simulink model "Tracking_01"  (R2022b)
settings: Solver=ode4  StartTime=0.0  StopTime=50  FixedStep=1e-3  MaxStep=1e-3  RelTol=1e-3
undefined symbols (not defined in the file or in its folder): OF_b, OF_k1, OF_k2, TT_theta1_init, TT_theta2_init, TT_theta3_init, TT_x_init, TT_y_init, v_sat, w_sat
libraries: simulink x18
settings Model: Creator=david  LastModifiedBy=emanuelevitetta

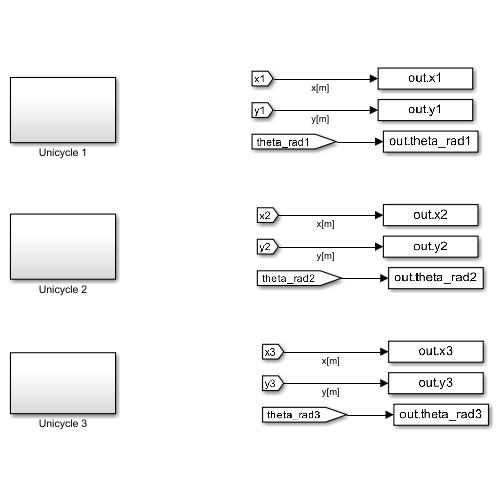
[thumbnail: Simulink's stored preview of the top-level diagram]
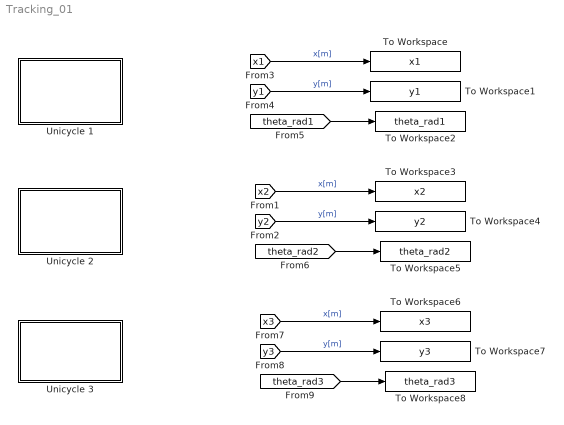
== system Tracking_01 ==
  To Workspace : ToWorkspace  VariableName=x1  SaveFormat=Structure With Time  SampleTime=-1
  To Workspace1 : ToWorkspace  VariableName=y1  SaveFormat=Structure With Time  SampleTime=-1
  To Workspace2 : ToWorkspace  VariableName=theta_rad1  SaveFormat=Structure With Time  SampleTime=-1
  To Workspace3 : ToWorkspace  VariableName=x2  SaveFormat=Structure With Time  SampleTime=-1
  To Workspace4 : ToWorkspace  VariableName=y2  SaveFormat=Structure With Time  SampleTime=-1
  To Workspace5 : ToWorkspace  VariableName=theta_rad2  SaveFormat=Structure With Time  SampleTime=-1
  To Workspace6 : ToWorkspace  VariableName=x3  SaveFormat=Structure With Time  SampleTime=-1
  To Workspace7 : ToWorkspace  VariableName=y3  SaveFormat=Structure With Time  SampleTime=-1
  To Workspace8 : ToWorkspace  VariableName=theta_rad3  SaveFormat=Structure With Time  SampleTime=-1
  Unicycle 1 : Subsystem
  Unicycle 2 : Subsystem
  Unicycle 3 : Subsystem
  wires:
  [x1] -> To Workspace/1  "x[m]"
  [y1] -> To Workspace1/1  "y[m]"
  [theta_rad1] -> To Workspace2/1
  [x2] -> To Workspace3/1  "x[m]"
  [y2] -> To Workspace4/1  "y[m]"
  [theta_rad2] -> To Workspace5/1
  [theta_rad3] -> To Workspace8/1
  [y3] -> To Workspace7/1  "y[m]"
  [x3] -> To Workspace6/1  "x[m]"

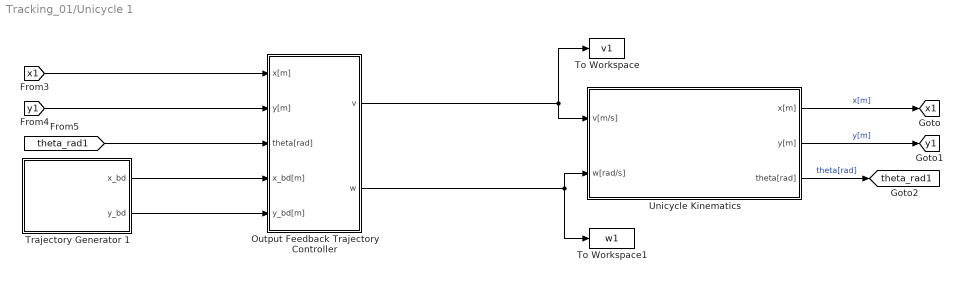
== system Tracking_01/Unicycle 1 ==
  Output Feedback Trajectory Controller : Subsystem
  To Workspace : ToWorkspace  VariableName=v1  SaveFormat=Structure With Time  SampleTime=-1
  To Workspace1 : ToWorkspace  VariableName=w1  SaveFormat=Structure With Time  SampleTime=-1
  Trajectory Generator 1 : Subsystem
  Unicycle Kinematics : Subsystem
  tag scope: theta_rad1=global, x1=global, y1=global
  wires:
  Unicycle Kinematics/3(theta[rad]) -> [theta_rad1]  "theta[rad]"
  Unicycle Kinematics/2(y[m]) -> [y1]  "y[m]"
  Unicycle Kinematics/1(x[m]) -> [x1]  "x[m]"
  [theta_rad1] -> Output Feedback Trajectory Controller/3(theta[rad])
  [x1] -> Output Feedback Trajectory Controller/1(x[m])
  [y1] -> Output Feedback Trajectory Controller/2(y[m])
  Trajectory Generator 1/1(x_bd) -> Output Feedback Trajectory Controller/4(x_bd[m])
  Trajectory Generator 1/2(y_bd) -> Output Feedback Trajectory Controller/5(y_bd[m])
  Output Feedback Trajectory Controller/2(w) -> Unicycle Kinematics/2(w[rad/s]), To Workspace1/1
  Output Feedback Trajectory Controller/1(v) -> To Workspace/1, Unicycle Kinematics/1(v[m/s])

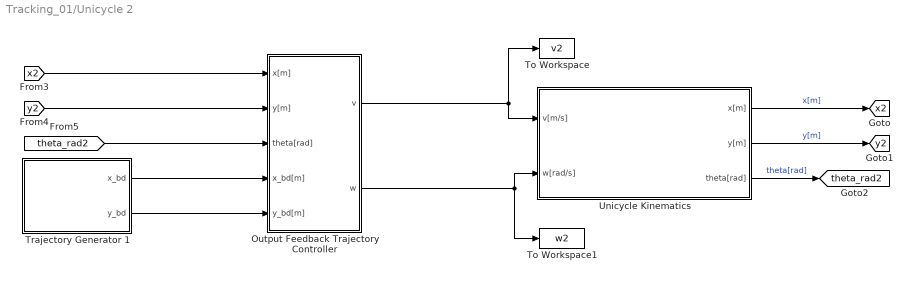
== system Tracking_01/Unicycle 2 ==
  Output Feedback Trajectory Controller : Subsystem
  To Workspace : ToWorkspace  VariableName=v2  SaveFormat=Structure With Time  SampleTime=-1
  To Workspace1 : ToWorkspace  VariableName=w2  SaveFormat=Structure With Time  SampleTime=-1
  Trajectory Generator 1 : Subsystem
  Unicycle Kinematics : Subsystem
  tag scope: theta_rad2=global, x2=global, y2=global
  wires:
  Unicycle Kinematics/3(theta[rad]) -> [theta_rad2]  "theta[rad]"
  Unicycle Kinematics/2(y[m]) -> [y2]  "y[m]"
  Unicycle Kinematics/1(x[m]) -> [x2]  "x[m]"
  [theta_rad2] -> Output Feedback Trajectory Controller/3(theta[rad])
  [x2] -> Output Feedback Trajectory Controller/1(x[m])
  [y2] -> Output Feedback Trajectory Controller/2(y[m])
  Trajectory Generator 1/1(x_bd) -> Output Feedback Trajectory Controller/4(x_bd[m])
  Trajectory Generator 1/2(y_bd) -> Output Feedback Trajectory Controller/5(y_bd[m])
  Output Feedback Trajectory Controller/2(w) -> Unicycle Kinematics/2(w[rad/s]), To Workspace1/1
  Output Feedback Trajectory Controller/1(v) -> Unicycle Kinematics/1(v[m/s]), To Workspace/1

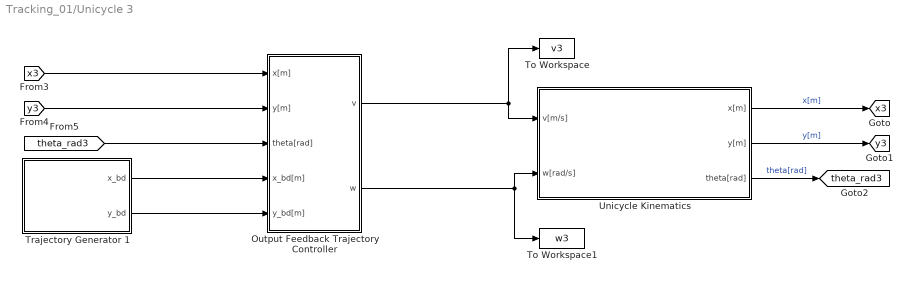
== system Tracking_01/Unicycle 3 ==
  Output Feedback Trajectory Controller : Subsystem
  To Workspace : ToWorkspace  VariableName=v3  SaveFormat=Structure With Time  SampleTime=-1
  To Workspace1 : ToWorkspace  VariableName=w3  SaveFormat=Structure With Time  SampleTime=-1
  Trajectory Generator 1 : Subsystem
  Unicycle Kinematics : Subsystem
  tag scope: theta_rad3=global, x3=global, y3=global
  wires:
  Unicycle Kinematics/3(theta[rad]) -> [theta_rad3]  "theta[rad]"
  Unicycle Kinematics/2(y[m]) -> [y3]  "y[m]"
  Unicycle Kinematics/1(x[m]) -> [x3]  "x[m]"
  [theta_rad3] -> Output Feedback Trajectory Controller/3(theta[rad])
  [x3] -> Output Feedback Trajectory Controller/1(x[m])
  [y3] -> Output Feedback Trajectory Controller/2(y[m])
  Trajectory Generator 1/1(x_bd) -> Output Feedback Trajectory Controller/4(x_bd[m])
  Trajectory Generator 1/2(y_bd) -> Output Feedback Trajectory Controller/5(y_bd[m])
  Output Feedback Trajectory Controller/2(w) -> Unicycle Kinematics/2(w[rad/s]), To Workspace1/1
  Output Feedback Trajectory Controller/1(v) -> Unicycle Kinematics/1(v[m/s]), To Workspace/1

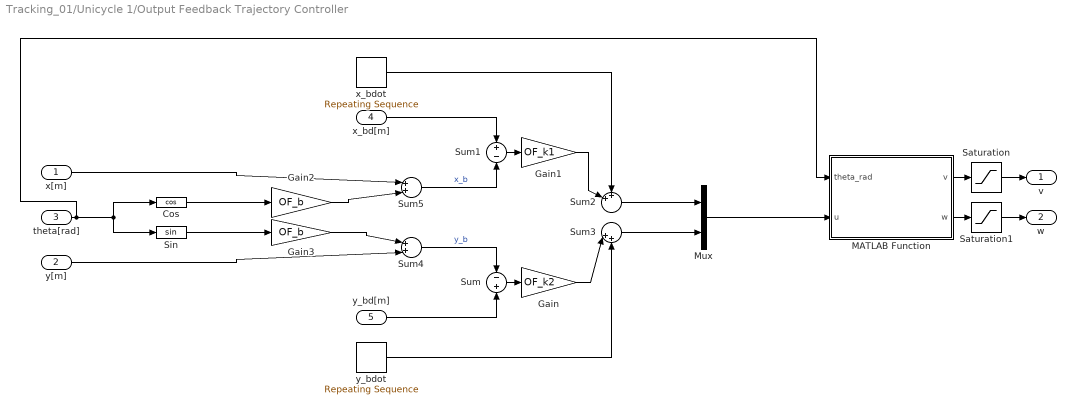
== system Tracking_01/Unicycle 1/Output Feedback Trajectory Controller ==
  x[m] : Inport
  y[m] : Inport  Port=2
  theta[rad] : Inport  Port=3
  x_bd[m] : Inport  Port=4
  y_bd[m] : Inport  Port=5
  Cos : Trigonometry  Operator=cos
  Gain : Gain  Gain=OF_k2
  Gain1 : Gain  Gain=OF_k1
  Gain2 : Gain  Gain=OF_b
  Gain3 : Gain  Gain=OF_b
  MATLAB Function : MATLAB Function  TreatAsAtomicUnit=on
  Mux : Mux  Inputs=2
  Saturation : Saturate  UpperLimit=v_sat  LowerLimit=-v_sat
  Saturation1 : Saturate  UpperLimit=w_sat  LowerLimit=-w_sat
  Sin : Trigonometry
  Sum : Sum  Inputs=-+
  Sum1 : Sum  Inputs=+-
  Sum2 : Sum  Inputs=++||
  Sum3 : Sum  Inputs=||++
  Sum4 : Sum  Inputs=|++|
  Sum5 : Sum  Inputs=|++|
  x_bdot : simulink/Sources/Repeating Sequence  rep_seq_t=time  rep_seq_y=x_bdot1
  y_bdot : simulink/Sources/Repeating Sequence  rep_seq_t=time  rep_seq_y=y_bdot1
  v : Outport
  w : Outport  Port=2
  wires:
  MATLAB Function/1(v) -> Saturation/1
  MATLAB Function/2(w) -> Saturation1/1
  x_bd[m]/1 -> Sum1/1
  y_bd[m]/1 -> Sum/2
  Mux/1 -> MATLAB Function/2(u)
  Sum2/1 -> Mux/1
  Sum3/1 -> Mux/2
  Sum/1 -> Gain/1
  Sum1/1 -> Gain1/1
  y_bdot/1 -> Sum3/2
  Gain/1 -> Sum3/1
  Gain1/1 -> Sum2/2
  x_bdot/1 -> Sum2/1
  Sum4/1 -> Sum/1  "y_b"
  Sum5/1 -> Sum1/2  "x_b"
  x[m]/1 -> Sum5/1
  y[m]/1 -> Sum4/2
  Cos/1 -> Gain2/1
  Gain3/1 -> Sum4/1
  Gain2/1 -> Sum5/2
  theta[rad]/1 -> Sin/1, Cos/1, MATLAB Function/1(theta_rad)
  Sin/1 -> Gain3/1
  Saturation/1 -> v/1
  Saturation1/1 -> w/1

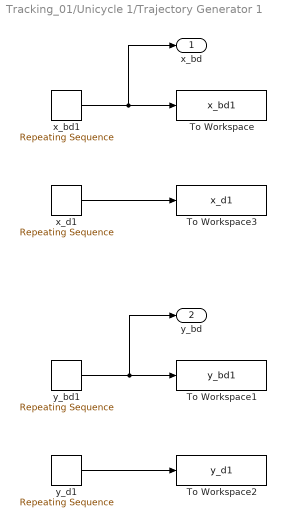
== system Tracking_01/Unicycle 1/Trajectory Generator 1 ==
  To Workspace : ToWorkspace  VariableName=x_bd1  SaveFormat=Structure With Time  SampleTime=-1
  To Workspace1 : ToWorkspace  VariableName=y_bd1  SaveFormat=Structure With Time  SampleTime=-1
  To Workspace2 : ToWorkspace  VariableName=y_d1  SaveFormat=Structure With Time  SampleTime=-1
  To Workspace3 : ToWorkspace  VariableName=x_d1  SaveFormat=Structure With Time  SampleTime=-1
  x_bd1 : simulink/Sources/Repeating Sequence  rep_seq_t=time  rep_seq_y=x_bd1
  x_d1 : simulink/Sources/Repeating Sequence  rep_seq_t=time  rep_seq_y=x_d1
  y_bd1 : simulink/Sources/Repeating Sequence  rep_seq_t=time  rep_seq_y=y_bd1
  y_d1 : simulink/Sources/Repeating Sequence  rep_seq_t=time  rep_seq_y=y_d1
  x_bd : Outport
  y_bd : Outport  Port=2
  wires:
  x_bd1/1 -> x_bd/1, To Workspace/1
  x_d1/1 -> To Workspace3/1
  y_bd1/1 -> y_bd/1, To Workspace1/1
  y_d1/1 -> To Workspace2/1

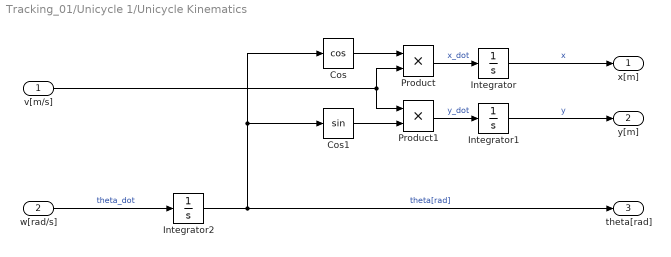
== system Tracking_01/Unicycle 1/Unicycle Kinematics ==
  v[m/s] : Inport
  w[rad/s] : Inport  Port=2
  Cos : Trigonometry  Operator=cos
  Cos1 : Trigonometry
  Integrator : Integrator  InitialCondition=TT_x_init
  Integrator1 : Integrator  InitialCondition=TT_y_init
  Integrator2 : Integrator  InitialCondition=TT_theta1_init
  Product : Product
  Product1 : Product
  x[m] : Outport
  y[m] : Outport  Port=2
  theta[rad] : Outport  Port=3
  wires:
  Integrator/1 -> x[m]/1  "x"
  Integrator1/1 -> y[m]/1  "y"
  w[rad/s]/1 -> Integrator2/1  "theta_dot"
  Integrator2/1 -> Cos/1, Cos1/1, theta[rad]/1  "theta[rad]"
  Product/1 -> Integrator/1  "x_dot"
  Cos1/1 -> Product1/2
  Cos/1 -> Product/1
  v[m/s]/1 -> Product1/1, Product/2
  Product1/1 -> Integrator1/1  "y_dot"

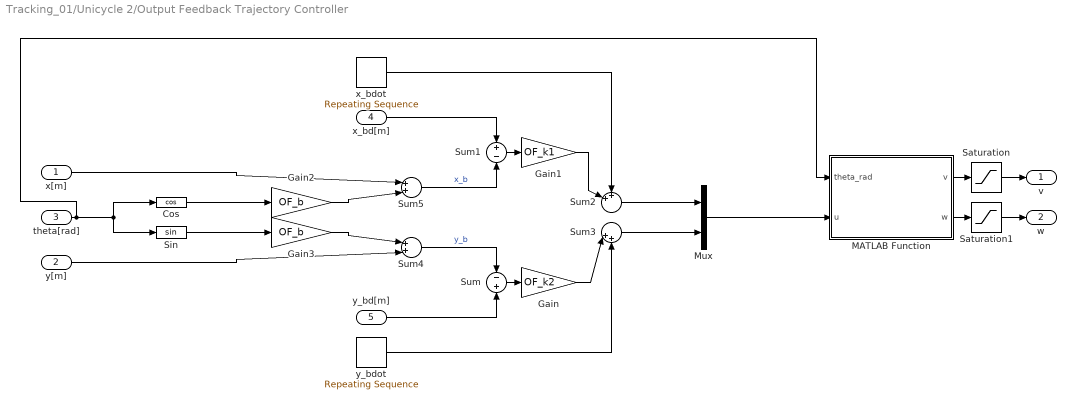
== system Tracking_01/Unicycle 2/Output Feedback Trajectory Controller ==
  x[m] : Inport
  y[m] : Inport  Port=2
  theta[rad] : Inport  Port=3
  x_bd[m] : Inport  Port=4
  y_bd[m] : Inport  Port=5
  Cos : Trigonometry  Operator=cos
  Gain : Gain  Gain=OF_k2
  Gain1 : Gain  Gain=OF_k1
  Gain2 : Gain  Gain=OF_b
  Gain3 : Gain  Gain=OF_b
  MATLAB Function : MATLAB Function  TreatAsAtomicUnit=on
  Mux : Mux  Inputs=2
  Saturation : Saturate  UpperLimit=v_sat  LowerLimit=-v_sat
  Saturation1 : Saturate  UpperLimit=w_sat  LowerLimit=-w_sat
  Sin : Trigonometry
  Sum : Sum  Inputs=-+
  Sum1 : Sum  Inputs=+-
  Sum2 : Sum  Inputs=++||
  Sum3 : Sum  Inputs=||++
  Sum4 : Sum  Inputs=|++|
  Sum5 : Sum  Inputs=|++|
  x_bdot : simulink/Sources/Repeating Sequence  rep_seq_t=time  rep_seq_y=x_bdot2
  y_bdot : simulink/Sources/Repeating Sequence  rep_seq_t=time  rep_seq_y=y_bdot2
  v : Outport
  w : Outport  Port=2
  wires:
  MATLAB Function/1(v) -> Saturation/1
  MATLAB Function/2(w) -> Saturation1/1
  x_bd[m]/1 -> Sum1/1
  y_bd[m]/1 -> Sum/2
  Mux/1 -> MATLAB Function/2(u)
  Sum2/1 -> Mux/1
  Sum3/1 -> Mux/2
  Sum/1 -> Gain/1
  Sum1/1 -> Gain1/1
  y_bdot/1 -> Sum3/2
  Gain/1 -> Sum3/1
  Gain1/1 -> Sum2/2
  x_bdot/1 -> Sum2/1
  Sum4/1 -> Sum/1  "y_b"
  Sum5/1 -> Sum1/2  "x_b"
  x[m]/1 -> Sum5/1
  y[m]/1 -> Sum4/2
  Cos/1 -> Gain2/1
  Gain3/1 -> Sum4/1
  Gain2/1 -> Sum5/2
  theta[rad]/1 -> Sin/1, Cos/1, MATLAB Function/1(theta_rad)
  Sin/1 -> Gain3/1
  Saturation1/1 -> w/1
  Saturation/1 -> v/1

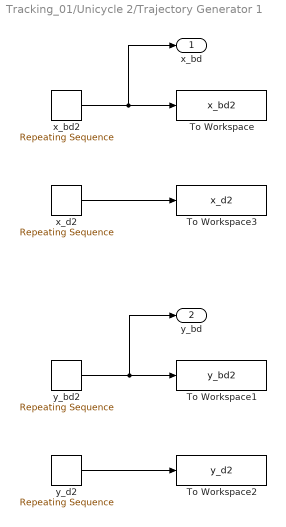
== system Tracking_01/Unicycle 2/Trajectory Generator 1 ==
  To Workspace : ToWorkspace  VariableName=x_bd2  SaveFormat=Structure With Time  SampleTime=-1
  To Workspace1 : ToWorkspace  VariableName=y_bd2  SaveFormat=Structure With Time  SampleTime=-1
  To Workspace2 : ToWorkspace  VariableName=y_d2  SaveFormat=Structure With Time  SampleTime=-1
  To Workspace3 : ToWorkspace  VariableName=x_d2  SaveFormat=Structure With Time  SampleTime=-1
  x_bd2 : simulink/Sources/Repeating Sequence  rep_seq_t=time  rep_seq_y=x_bd2
  x_d2 : simulink/Sources/Repeating Sequence  rep_seq_t=time  rep_seq_y=x_d2
  y_bd2 : simulink/Sources/Repeating Sequence  rep_seq_t=time  rep_seq_y=y_bd2
  y_d2 : simulink/Sources/Repeating Sequence  rep_seq_t=time  rep_seq_y=y_d2
  x_bd : Outport
  y_bd : Outport  Port=2
  wires:
  x_bd2/1 -> x_bd/1, To Workspace/1
  x_d2/1 -> To Workspace3/1
  y_bd2/1 -> y_bd/1, To Workspace1/1
  y_d2/1 -> To Workspace2/1

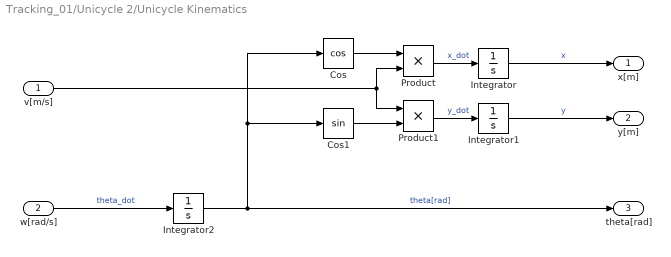
== system Tracking_01/Unicycle 2/Unicycle Kinematics ==
  v[m/s] : Inport
  w[rad/s] : Inport  Port=2
  Cos : Trigonometry  Operator=cos
  Cos1 : Trigonometry
  Integrator : Integrator  InitialCondition=TT_x_init
  Integrator1 : Integrator  InitialCondition=TT_y_init
  Integrator2 : Integrator  InitialCondition=TT_theta2_init
  Product : Product
  Product1 : Product
  x[m] : Outport
  y[m] : Outport  Port=2
  theta[rad] : Outport  Port=3
  wires:
  Integrator/1 -> x[m]/1  "x"
  Integrator1/1 -> y[m]/1  "y"
  w[rad/s]/1 -> Integrator2/1  "theta_dot"
  Integrator2/1 -> Cos/1, Cos1/1, theta[rad]/1  "theta[rad]"
  Product/1 -> Integrator/1  "x_dot"
  Cos1/1 -> Product1/2
  Cos/1 -> Product/1
  v[m/s]/1 -> Product1/1, Product/2
  Product1/1 -> Integrator1/1  "y_dot"

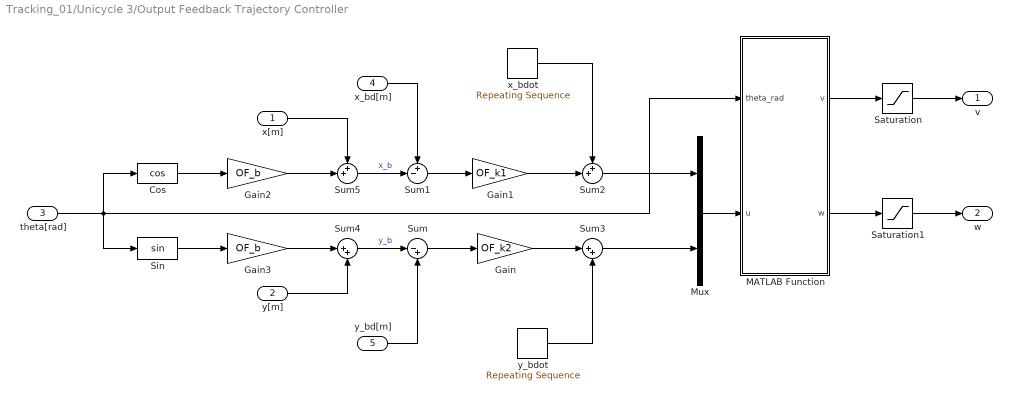
== system Tracking_01/Unicycle 3/Output Feedback Trajectory Controller ==
  x[m] : Inport
  y[m] : Inport  Port=2
  theta[rad] : Inport  Port=3
  x_bd[m] : Inport  Port=4
  y_bd[m] : Inport  Port=5
  Cos : Trigonometry  Operator=cos
  Gain : Gain  Gain=OF_k2
  Gain1 : Gain  Gain=OF_k1
  Gain2 : Gain  Gain=OF_b
  Gain3 : Gain  Gain=OF_b
  MATLAB Function : MATLAB Function  TreatAsAtomicUnit=on
  Mux : Mux  Inputs=2
  Saturation : Saturate  UpperLimit=v_sat  LowerLimit=-v_sat
  Saturation1 : Saturate  UpperLimit=w_sat  LowerLimit=-w_sat
  Sin : Trigonometry
  Sum : Sum  Inputs=|-+
  Sum1 : Sum  Inputs=+-|
  Sum2 : Sum  Inputs=++|
  Sum3 : Sum  Inputs=|++
  Sum4 : Sum  Inputs=|++
  Sum5 : Sum  Inputs=++|
  x_bdot : simulink/Sources/Repeating Sequence  rep_seq_t=time  rep_seq_y=x_bdot3
  y_bdot : simulink/Sources/Repeating Sequence  rep_seq_t=time  rep_seq_y=y_bdot3
  v : Outport
  w : Outport  Port=2
  wires:
  MATLAB Function/1(v) -> Saturation/1
  MATLAB Function/2(w) -> Saturation1/1
  x_bd[m]/1 -> Sum1/1
  y_bd[m]/1 -> Sum/2
  Mux/1 -> MATLAB Function/2(u)
  Sum2/1 -> Mux/1
  Sum3/1 -> Mux/2
  Sum/1 -> Gain/1
  Sum1/1 -> Gain1/1
  y_bdot/1 -> Sum3/2
  Gain/1 -> Sum3/1
  Gain1/1 -> Sum2/2
  x_bdot/1 -> Sum2/1
  Sum4/1 -> Sum/1  "y_b"
  Sum5/1 -> Sum1/2  "x_b"
  x[m]/1 -> Sum5/1
  y[m]/1 -> Sum4/2
  Cos/1 -> Gain2/1
  Gain3/1 -> Sum4/1
  Gain2/1 -> Sum5/2
  theta[rad]/1 -> Sin/1, Cos/1, MATLAB Function/1(theta_rad)
  Sin/1 -> Gain3/1
  Saturation/1 -> v/1
  Saturation1/1 -> w/1

== system Tracking_01/Unicycle 3/Trajectory Generator 1 ==
  To Workspace : ToWorkspace  VariableName=x_bd3  SaveFormat=Structure With Time  SampleTime=-1
  To Workspace1 : ToWorkspace  VariableName=y_bd3  SaveFormat=Structure With Time  SampleTime=-1
  To Workspace2 : ToWorkspace  VariableName=y_d3  SaveFormat=Structure With Time  SampleTime=-1
  To Workspace3 : ToWorkspace  VariableName=x_d3  SaveFormat=Structure With Time  SampleTime=-1
  x_bd3 : simulink/Sources/Repeating Sequence  rep_seq_t=time  rep_seq_y=x_bd3
  x_d3 : simulink/Sources/Repeating Sequence  rep_seq_t=time  rep_seq_y=x_d3
  y_bd3 : simulink/Sources/Repeating Sequence  rep_seq_t=time  rep_seq_y=y_bd3
  y_d3 : simulink/Sources/Repeating Sequence  rep_seq_t=time  rep_seq_y=y_d3
  x_bd : Outport
  y_bd : Outport  Port=2
  wires:
  x_bd3/1 -> x_bd/1, To Workspace/1
  x_d3/1 -> To Workspace3/1
  y_bd3/1 -> y_bd/1, To Workspace1/1
  y_d3/1 -> To Workspace2/1

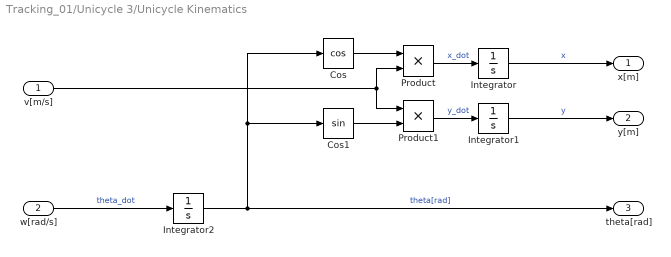
== system Tracking_01/Unicycle 3/Unicycle Kinematics ==
  v[m/s] : Inport
  w[rad/s] : Inport  Port=2
  Cos : Trigonometry  Operator=cos
  Cos1 : Trigonometry
  Integrator : Integrator  InitialCondition=TT_x_init
  Integrator1 : Integrator  InitialCondition=TT_y_init
  Integrator2 : Integrator  InitialCondition=TT_theta3_init
  Product : Product
  Product1 : Product
  x[m] : Outport
  y[m] : Outport  Port=2
  theta[rad] : Outport  Port=3
  wires:
  Integrator/1 -> x[m]/1  "x"
  Integrator1/1 -> y[m]/1  "y"
  w[rad/s]/1 -> Integrator2/1  "theta_dot"
  Integrator2/1 -> Cos/1, Cos1/1, theta[rad]/1  "theta[rad]"
  Product/1 -> Integrator/1  "x_dot"
  Cos1/1 -> Product1/2
  Cos/1 -> Product/1
  v[m/s]/1 -> Product1/1, Product/2
  Product1/1 -> Integrator1/1  "y_dot"

== matlab function Tracking_01/Unicycle 2/Output Feedback Trajectory Controller/MATLAB Function ==
  data: theta_rad input; u input; v output; w output; OF_b parameter
function [v,w] = fcn(theta_rad, u, OF_b)


T_inv=[cos(theta_rad)       sin(theta_rad);
       -sin(theta_rad)/OF_b    cos(theta_rad)/OF_b];

in=T_inv*u;

v = in(1);
w= in(2);

== matlab function Tracking_01/Unicycle 1/Output Feedback Trajectory Controller/MATLAB Function ==
  data: theta_rad input; u input; v output; w output; OF_b parameter
function [v,w] = fcn(theta_rad, u, OF_b)


T_inv=[cos(theta_rad)       sin(theta_rad);
       -sin(theta_rad)/OF_b    cos(theta_rad)/OF_b];

in=T_inv*u;

v = in(1);
w= in(2);

== matlab function Tracking_01/Unicycle 3/Output Feedback Trajectory Controller/MATLAB Function ==
  data: theta_rad input; u input; v output; w output; OF_b parameter
function [v,w] = fcn(theta_rad, u, OF_b)


T_inv=[cos(theta_rad)       sin(theta_rad);
       -sin(theta_rad)/OF_b    cos(theta_rad)/OF_b];

in=T_inv*u;

v = in(1);
w= in(2);
